simulink model "RoboBoatVU_2014_Athena"  (R2014a)
settings: Solver=FixedStepDiscrete  StartTime=0.0  StopTime=inf  FixedStep=.1  RelTol=1e-3
undefined symbols (not defined in the file): Com1, Com2, Com3, Com4, DiscIntNeverNeededParam, RGB24, standard, strel
libraries: visiontextngfix x25, dspmtrx3 x22, simulink x19, xpcseriallib x12, slrtlib x7, speedgoatlib_IO102 x6, dspstat3 x5, visionstatistics x3, dspindex x2, xpcvideousblib x2, xpcvideoutillib x2, visionmorphops x1
(part 1 of 4)
settings Model: BufferReuse=off  Creator=wildcat  LastModifiedBy=Villanova ASV
settings SolverCC: EnableConcurrentExecution=on
settings DataIOCC: SignalLoggingSaveFormat=ModelDataLogs
settings OptimizationCC: BlockReduction=off  OptimizeBlockIOStorage=off  BufferReuse=off  GlobalBufferReuse=off  ExpressionFolding=off  LocalBlockOutputs=off
settings DebuggingCC: UnderspecifiedInitializationDetection=Classic  StateNameClashWarn=warning
settings HardwareCC: ProdIntDivRoundTo=Zero  ProdEndianess=LittleEndian  ProdHWDeviceType=Generic->32-bit x86 compatible
settings RTWCC: SystemTargetFile=slrt.tlc  TemplateMakefile=slrt_default_tmf  Description=Simulink Real-Time  ProcessScript=slrt_make_rtw_hook  RTWCompilerOptimization=On
settings SimulinkRealTimeCC: GeneratePreprocessorConditionals=Disable all  EnableShiftOperators=on

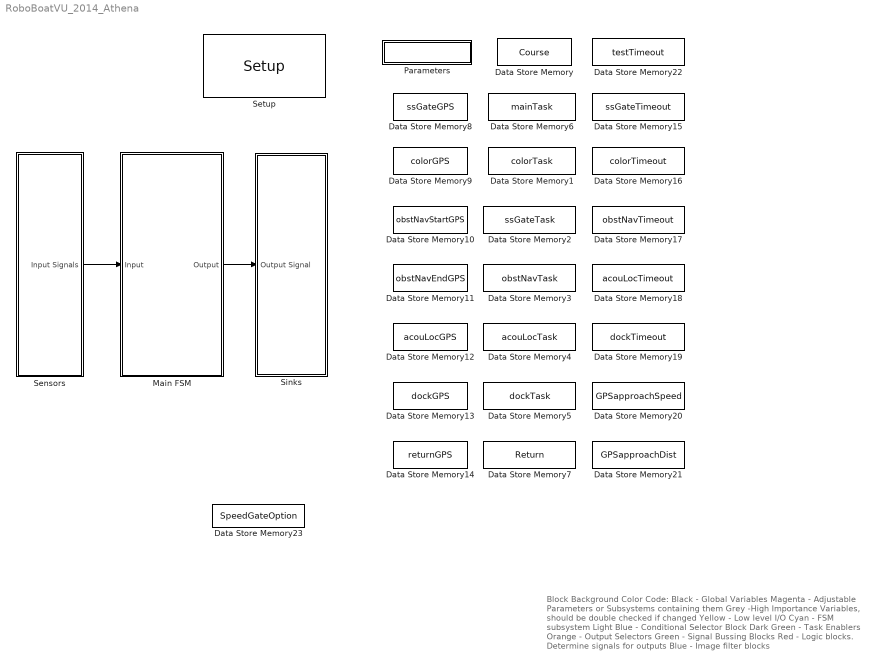
== system RoboBoatVU_2014_Athena ==
  note: Block Background Color Code:
      | Black - Global Variables
      | Magenta - Adjustable Parameters or Subsystems containing them
      | Grey -High Importance Variables, should be double checked if changed
      | Yellow - Low level I/O
      | Cyan - FSM subsystem
      | Light Blue - Conditional Selector Block
      | Dark Green - Task Enablers
      | Orange - Output Selectors
      | Green - Signal Bussing Blocks
      | Red - Logic blocks. Determine signals for outputs
      | Blue - Image filter blocks
  Data Store Memory : DataStoreMemory  DataStoreName=Course  ReadBeforeWriteMsg=warning  WriteAfterWriteMsg=warning  WriteAfterReadMsg=warning
  Data Store Memory1 : DataStoreMemory  DataStoreName=colorTask  ReadBeforeWriteMsg=warning  WriteAfterWriteMsg=warning  WriteAfterReadMsg=warning  InitialValue=zeros(1,8)
  Data Store Memory10 : DataStoreMemory  DataStoreName=obstNavStartGPS  ReadBeforeWriteMsg=warning  WriteAfterWriteMsg=warning  WriteAfterReadMsg=warning  InitialValue=zeros(1,2)
  Data Store Memory11 : DataStoreMemory  DataStoreName=obstNavEndGPS  ReadBeforeWriteMsg=warning  WriteAfterWriteMsg=warning  WriteAfterReadMsg=warning  InitialValue=zeros(1,2)
  Data Store Memory12 : DataStoreMemory  DataStoreName=acouLocGPS  ReadBeforeWriteMsg=warning  WriteAfterWriteMsg=warning  WriteAfterReadMsg=warning  InitialValue=zeros(1,2)
  Data Store Memory13 : DataStoreMemory  DataStoreName=dockGPS  ReadBeforeWriteMsg=warning  WriteAfterWriteMsg=warning  WriteAfterReadMsg=warning  InitialValue=zeros(1,2)
  Data Store Memory14 : DataStoreMemory  DataStoreName=returnGPS  ReadBeforeWriteMsg=warning  WriteAfterWriteMsg=warning  WriteAfterReadMsg=warning  InitialValue=zeros(1,2)
  Data Store Memory15 : DataStoreMemory  DataStoreName=ssGateTimeout  ReadBeforeWriteMsg=warning  WriteAfterWriteMsg=warning  WriteAfterReadMsg=warning
  Data Store Memory16 : DataStoreMemory  DataStoreName=colorTimeout  ReadBeforeWriteMsg=warning  WriteAfterWriteMsg=warning  WriteAfterReadMsg=warning
  Data Store Memory17 : DataStoreMemory  DataStoreName=obstNavTimeout  ReadBeforeWriteMsg=warning  WriteAfterWriteMsg=warning  WriteAfterReadMsg=warning
  Data Store Memory18 : DataStoreMemory  DataStoreName=acouLocTimeout  ReadBeforeWriteMsg=warning  WriteAfterWriteMsg=warning  WriteAfterReadMsg=warning
  Data Store Memory19 : DataStoreMemory  DataStoreName=dockTimeout  ReadBeforeWriteMsg=warning  WriteAfterWriteMsg=warning  WriteAfterReadMsg=warning
  Data Store Memory2 : DataStoreMemory  DataStoreName=ssGateTask  ReadBeforeWriteMsg=warning  WriteAfterWriteMsg=warning  WriteAfterReadMsg=warning  InitialValue=zeros(1,8)
  Data Store Memory20 : DataStoreMemory  DataStoreName=GPSapproachSpeed  ReadBeforeWriteMsg=warning  WriteAfterWriteMsg=warning  WriteAfterReadMsg=warning
  Data Store Memory21 : DataStoreMemory  DataStoreName=GPSapproachDist  ReadBeforeWriteMsg=warning  WriteAfterWriteMsg=warning  WriteAfterReadMsg=warning
  Data Store Memory22 : DataStoreMemory  DataStoreName=testTimeout  ReadBeforeWriteMsg=warning  WriteAfterWriteMsg=warning  WriteAfterReadMsg=warning
  Data Store Memory23 : DataStoreMemory  DataStoreName=SpeedGateOption  ReadBeforeWriteMsg=warning  WriteAfterWriteMsg=warning  WriteAfterReadMsg=warning  InitialValue=zeros(1,8)
  Data Store Memory3 : DataStoreMemory  DataStoreName=obstNavTask  ReadBeforeWriteMsg=warning  WriteAfterWriteMsg=warning  WriteAfterReadMsg=warning  InitialValue=zeros(1,8)
  Data Store Memory4 : DataStoreMemory  DataStoreName=acouLocTask  ReadBeforeWriteMsg=warning  WriteAfterWriteMsg=warning  WriteAfterReadMsg=warning  InitialValue=zeros(1,8)
  Data Store Memory5 : DataStoreMemory  DataStoreName=dockTask  ReadBeforeWriteMsg=warning  WriteAfterWriteMsg=warning  WriteAfterReadMsg=warning  InitialValue=zeros(1,8)
  Data Store Memory6 : DataStoreMemory  DataStoreName=mainTask  ReadBeforeWriteMsg=warning  WriteAfterWriteMsg=warning  WriteAfterReadMsg=warning  InitialValue=zeros(1,8)
  Data Store Memory7 : DataStoreMemory  DataStoreName=Return  ReadBeforeWriteMsg=warning  WriteAfterWriteMsg=warning  WriteAfterReadMsg=warning  InitialValue=zeros(1,8)
  Data Store Memory8 : DataStoreMemory  DataStoreName=ssGateGPS  ReadBeforeWriteMsg=warning  WriteAfterWriteMsg=warning  WriteAfterReadMsg=warning  InitialValue=zeros(1,2)
  Data Store Memory9 : DataStoreMemory  DataStoreName=colorGPS  ReadBeforeWriteMsg=warning  WriteAfterWriteMsg=warning  WriteAfterReadMsg=warning  InitialValue=zeros(1,2)
  Main FSM : Subsystem
  Parameters : Subsystem
  Sensors : Subsystem
  Setup : speedgoatlib_IO102/Setup  group=Digital output setup  id=1  range=+-5V  cal=off  pciSlot=-1  adChannelMode=Multiple-channel (enter number of channels below)  adChannel=16  adCoupling=Differential  daChannel=[1,2,3,4]  daReset=[1]  daInitValue=[0]  diChannel=[1,2,3,4,5,6,7,8]  doChannel=[1,2,3,4,5,6,7,8]  doReset=[1]  doInitValue=[0]
  Sinks : Subsystem
  wires:
  Main FSM/1(Output) -> Sinks/1(Output Signal)
  Sensors/1(Input Signals) -> Main FSM/1(Input)

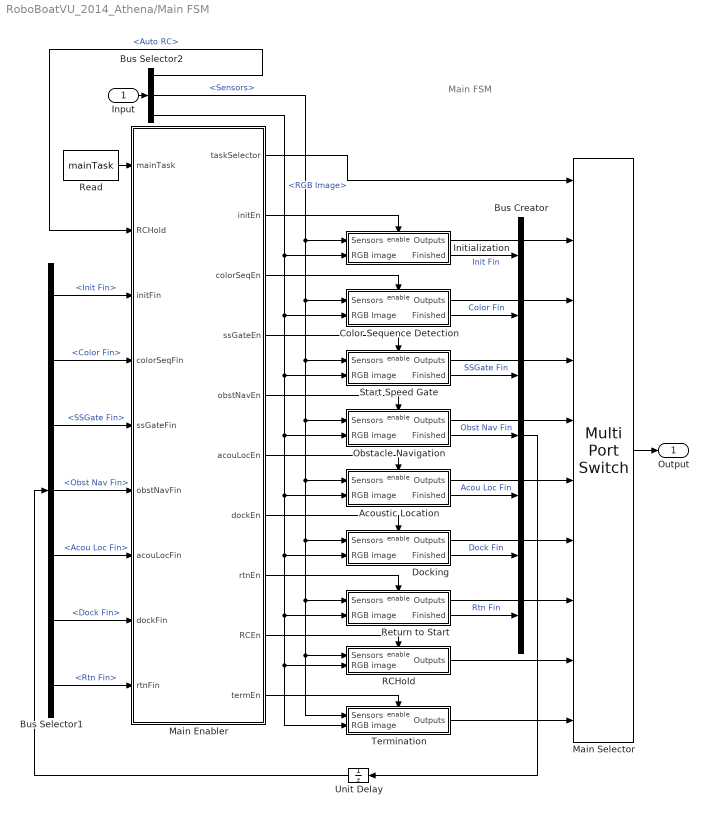
== system RoboBoatVU_2014_Athena/Main FSM ==
  note: Main FSM
  Input : Inport
  Acoustic Location : Subsystem  TreatAsAtomicUnit=on
  Bus Creator : BusCreator  Inputs=7
  Bus Selector1 : BusSelector  OutputSignals=Init Fin,Color Fin,SSGate Fin,Obst Nav Fin,Acou Loc Fin,Dock Fin,Rtn Fin
  Bus Selector2 : BusSelector  OutputSignals=Sensors.Digital In.Auto RC,Sensors,RGB Image
  Color Sequence Detection : Subsystem  TreatAsAtomicUnit=on
  Docking : Subsystem  TreatAsAtomicUnit=on
  Initialization : Subsystem
  Main Enabler : MATLAB Function  TreatAsAtomicUnit=on
  Main Selector : MultiPortSwitch  Inputs=9
  Obstacle Navigation : Subsystem  TreatAsAtomicUnit=on
  RCHold : Subsystem
  Read : DataStoreRead  DataStoreName=mainTask  SampleTime=0.1
  Return to Start : Subsystem  TreatAsAtomicUnit=on
  Start Speed Gate : Subsystem  TreatAsAtomicUnit=on
  Termination : Subsystem  TreatAsAtomicUnit=on
  Unit Delay : UnitDelay  SampleTime=-1
  Output : Outport
  wires:
  Bus Creator/1 -> Unit Delay/1
  Initialization/1(Outputs) -> Main Selector/2
  Main Selector/1 -> Output/1
  Read/1 -> Main Enabler/1(mainTask)
  Main Enabler/1(taskSelector) -> Main Selector/1
  Initialization/2(Finished) -> Bus Creator/1  "Init Fin"
  Unit Delay/1 -> Bus Selector1/1
  Input/1 -> Bus Selector2/1
  Bus Selector2/1 -> Main Enabler/2(RCHold)  "<Auto RC>"
  Main Enabler/2(initEn) -> Initialization/Enable
  Termination/1(Outputs) -> Main Selector/10
  RCHold/1(Outputs) -> Main Selector/9
  Main Enabler/9(RCEn) -> RCHold/Enable
  Main Enabler/10(termEn) -> Termination/Enable
  Bus Selector2/2 -> Initialization/1(Sensors), Color Sequence Detection/1(Sensors), Start Speed Gate/1(Sensors), Obstacle Navigation/1(Sensors), Docking/1(Sensors), Return to Start/1(Sensors), RCHold/1(Sensors), Termination/1(Sensors), Acoustic Location/1(Sensors)  "<Sensors>"
  Bus Selector2/3 -> Initialization/2(RGB image), Color Sequence Detection/2(RGB Image), Start Speed Gate/2(RGB image), Obstacle Navigation/2(RGB image), Docking/2(RGB image), Return to Start/2(RGB image), Termination/2(RGB image), RCHold/2(RGB image), Acoustic Location/2(RGB image)  "<RGB Image>"
  Color Sequence Detection/2(Finished) -> Bus Creator/2  "Color Fin"
  Start Speed Gate/2(Finished) -> Bus Creator/3  "SSGate Fin"
  Obstacle Navigation/2(Finished) -> Bus Creator/4  "Obst Nav Fin"
  Acoustic Location/2(Finished) -> Bus Creator/5  "Acou Loc Fin"
  Docking/2(Finished) -> Bus Creator/6  "Dock Fin"
  Return to Start/2(Finished) -> Bus Creator/7  "Rtn Fin"
  Return to Start/1(Outputs) -> Main Selector/8
  Docking/1(Outputs) -> Main Selector/7
  Acoustic Location/1(Outputs) -> Main Selector/6
  Obstacle Navigation/1(Outputs) -> Main Selector/5
  Start Speed Gate/1(Outputs) -> Main Selector/4
  Color Sequence Detection/1(Outputs) -> Main Selector/3
  Main Enabler/3(colorSeqEn) -> Color Sequence Detection/Enable
  Main Enabler/5(obstNavEn) -> Obstacle Navigation/Enable
  Main Enabler/6(acouLocEn) -> Acoustic Location/Enable
  Main Enabler/7(dockEn) -> Docking/Enable
  Main Enabler/8(rtnEn) -> Return to Start/Enable
  Bus Selector1/6 -> Main Enabler/8(dockFin)  "<Dock Fin>"
  Bus Selector1/1 -> Main Enabler/3(initFin)  "<Init Fin>"
  Bus Selector1/4 -> Main Enabler/6(obstNavFin)  "<Obst Nav Fin>"
  Bus Selector1/5 -> Main Enabler/7(acouLocFin)  "<Acou Loc Fin>"
  Bus Selector1/2 -> Main Enabler/4(colorSeqFin)  "<Color Fin>"
  Bus Selector1/3 -> Main Enabler/5(ssGateFin)  "<SSGate Fin>"
  Bus Selector1/7 -> Main Enabler/9(rtnFin)  "<Rtn Fin>"
  Main Enabler/4(ssGateEn) -> Start Speed Gate/Enable

== system RoboBoatVU_2014_Athena/Parameters ==
  note: Course options are:
      | A, B and
      | otherwise (for testing,
      |  must be one character)
  CourseName : Constant  Value=uint8('T')  VectorParams1D=off
  GPS Points : Subsystem
  Task Options : Subsystem
  Task Selector : Subsystem
  Timeouts and Constants : Subsystem
  Write : DataStoreWrite  DataStoreName=Course
  wires:
  CourseName/1 -> Write/1

== system RoboBoatVU_2014_Athena/Sensors ==
  Analog In : Subsystem
  Bus Creator : BusCreator  Inputs=2
  Bus Creator1 : BusCreator  Inputs=2
  Digital In : Subsystem
  Serial In : Subsystem
  Video In : Subsystem
  Input Signals : Outport
  wires:
  Serial In/1(Serial In) -> Bus Creator/1
  Digital In/1(Digital In) -> Bus Creator/2
  Video In/1(RGB image) -> Bus Creator1/2
  Bus Creator/1 -> Bus Creator1/1  "Sensors"
  Bus Creator1/1 -> Input Signals/1

== system RoboBoatVU_2014_Athena/Sinks ==
  Output Signal : Inport
  Bus Selector : BusSelector  OutputSignals=Sensors.Serial In.Compass.Heading,Outputs.Control Signals,Outputs.Annotated Image,Outputs.Control Signals.Arduino Signals
  Digital Outputs : Subsystem
  Image Transmission : Subsystem
  actuators : Subsystem
  data log : Subsystem  Commented=on
  wires:
  Bus Selector/2 -> actuators/2(Control Signals)  "<Control Signals>"
  Bus Selector/3 -> Image Transmission/1(RGB Image)  "<Annotated Image>"
  Bus Selector/1 -> actuators/1(Compass Heading)  "<Heading>"
  Output Signal/1 -> data log/1(Output signal), Bus Selector/1
  Bus Selector/4 -> Digital Outputs/1(Digital Outputs)  "<Arduino Signals>"

== system RoboBoatVU_2014_Athena/Main FSM/Acoustic Location ==
  note: Acoustic Location
  Sensors : Inport
  RGB image : Inport  Port=2
  Enable : EnablePort
  Bus Creator : BusCreator
  Bus Selector : BusSelector  OutputSignals=Mid S Fin,Left T Fin,Left S Fin,Right T Fin
  Bus Selector1 : BusSelector  OutputSignals=Output Signals,Task Finished
  Left Sample : Subsystem  TreatAsAtomicUnit=on
  Left Turn : Subsystem  TreatAsAtomicUnit=on
  MATLAB Function : MATLAB Function  TreatAsAtomicUnit=on
  Mid Sample : Subsystem  TreatAsAtomicUnit=on
  Multiport Switch : MultiPortSwitch  Inputs=5
  Right Sample : Subsystem  TreatAsAtomicUnit=on
  Right Turn : Subsystem  TreatAsAtomicUnit=on
  Unit Delay : UnitDelay  SampleTime=-1
  Outputs : Outport
  Finished : Outport  Port=2
  wires:
  Sensors/1 -> Left Turn/1(Sensors), Left Sample/1(Sensors), Right Turn/1(Sensors), Right Sample/1(Sensors), Mid Sample/1(Sensors)
  RGB image/1 -> Mid Sample/2(RGB Image), Left Turn/2(RGB Image), Right Turn/2(RGB Image), Right Sample/2(RGB Image), Left Sample/2(RGB Image)
  MATLAB Function/1(taskSelector) -> Multiport Switch/1
  MATLAB Function/2(midSampleEn) -> Mid Sample/Enable
  MATLAB Function/3(leftTurnEn) -> Left Turn/Enable
  MATLAB Function/4(leftSampleEn) -> Left Sample/Enable
  MATLAB Function/5(rightTurnEn) -> Right Turn/Enable
  MATLAB Function/6(rightSampleEn) -> Right Sample/Enable
  Mid Sample/1(Outputs) -> Multiport Switch/2
  Left Turn/1(Outputs) -> Multiport Switch/3
  Left Sample/1(Outputs) -> Multiport Switch/4
  Right Turn/1(Outputs) -> Multiport Switch/5
  Right Sample/1(Outputs) -> Multiport Switch/6
  Mid Sample/2(Finished) -> Bus Creator/1  "Mid S Fin"
  Left Turn/2(Finished) -> Bus Creator/2  "Left T Fin"
  Left Sample/2(Finished) -> Bus Creator/3  "Left S Fin"
  Right Turn/2(Finished) -> Bus Creator/4  "Right T Fin"
  Bus Creator/1 -> Unit Delay/1
  Unit Delay/1 -> Bus Selector/1
  Bus Selector/1 -> MATLAB Function/1(midSampleFin)  "<Mid S Fin>"
  Bus Selector/4 -> MATLAB Function/4(rightTurnFin)  "<Right T Fin>"
  Bus Selector/2 -> MATLAB Function/2(leftTurnFin)  "<Left T Fin>"
  Bus Selector/3 -> MATLAB Function/3(leftSampleFin)  "<Left S Fin>"
  Multiport Switch/1 -> Bus Selector1/1
  Bus Selector1/2 -> Finished/1  "<Task Finished>"
  Bus Selector1/1 -> Outputs/1  "<Output Signals>"

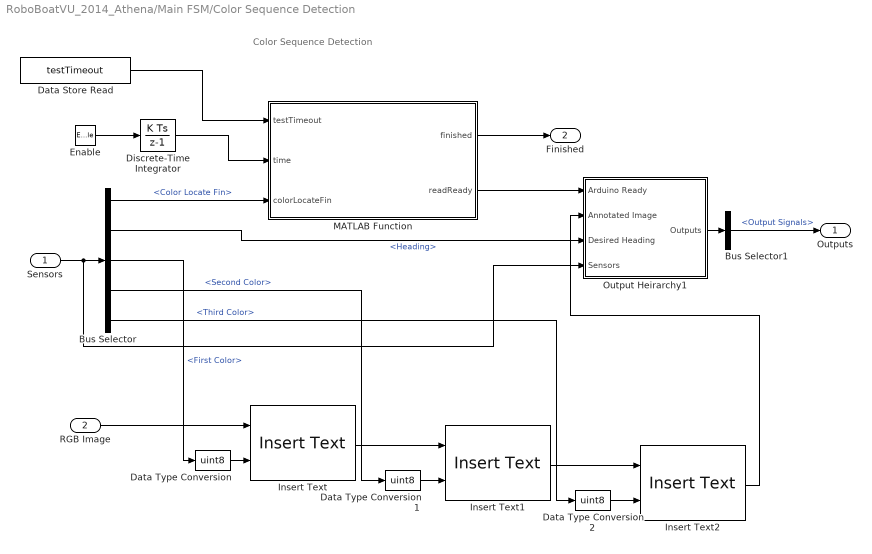
== system RoboBoatVU_2014_Athena/Main FSM/Color Sequence Detection ==
  note: Color Sequence Detection
  Sensors : Inport
  RGB Image : Inport  Port=2
  Enable : EnablePort  ShowOutputPort=on
  Bus Selector : BusSelector  OutputSignals=Digital In.Color Locate Fin,Serial In.Compass.Heading,Serial In.Arduino Messages.First Color,Serial In.Arduino Messages.Second Color,Serial In.Arduino Messages.Third Color
  Bus Selector1 : BusSelector  OutputSignals=Output Signals
  Data Store Read : DataStoreRead  DataStoreName=testTimeout
  Data Type Conversion : DataTypeConversion  OutDataTypeStr=uint8
  Data Type Conversion1 : DataTypeConversion  OutDataTypeStr=uint8
  Data Type Conversion2 : DataTypeConversion  OutDataTypeStr=uint8
  Discrete-Time Integrator : DiscreteIntegrator  SampleTime=0.1  ICPrevOutput=DiscIntNeverNeededParam  ICPrevScaledInput=DiscIntNeverNeededParam
  Insert Text : visiontextngfix/Insert Text  inputType=Obsolete  theText='First Color: %d'  getTextLocFrom=Specify via dialog  textLoc=[1 1]  getTextColorFrom=Specify via dialog  textColor=[0 0 0]  getTextIntensityFrom=Specify via dialog  textIntensity=0  getTextOpacityFrom=Specify via dialog  textOpacity=1.0  dummyVar2=0  dummyVar3=0  dummyVar4=0  imagePorts=One multidimensional signal  isInputTransposed=off  fontFace=LucidaSansRegular  dummyVar1=0  blockFontSize=12  antiAliased=on
  Insert Text1 : visiontextngfix/Insert Text  inputType=Obsolete  theText='Second Color: %d'  getTextLocFrom=Specify via dialog  textLoc=[1 10]  getTextColorFrom=Specify via dialog  textColor=[0 0 0]  getTextIntensityFrom=Specify via dialog  textIntensity=0  getTextOpacityFrom=Specify via dialog  textOpacity=1.0  dummyVar2=0  dummyVar3=0  dummyVar4=0  imagePorts=One multidimensional signal  isInputTransposed=off  fontFace=LucidaSansRegular  dummyVar1=0  blockFontSize=12  antiAliased=on
  Insert Text2 : visiontextngfix/Insert Text  inputType=Obsolete  theText='Third Color: %d'  getTextLocFrom=Specify via dialog  textLoc=[1 20]  getTextColorFrom=Specify via dialog  textColor=[0 0 0]  getTextIntensityFrom=Specify via dialog  textIntensity=0  getTextOpacityFrom=Specify via dialog  textOpacity=1.0  dummyVar2=0  dummyVar3=0  dummyVar4=0  imagePorts=One multidimensional signal  isInputTransposed=off  fontFace=LucidaSansRegular  dummyVar1=0  blockFontSize=12  antiAliased=on
  MATLAB Function : MATLAB Function  TreatAsAtomicUnit=on
  Output Heirarchy1 : Subsystem
  Outputs : Outport
  Finished : Outport  Port=2
  wires:
  Sensors/1 -> Output Heirarchy1/4(Sensors), Bus Selector/1
  Bus Selector/1 -> MATLAB Function/3(colorLocateFin)  "<Color Locate Fin>"
  MATLAB Function/2(readReady) -> Output Heirarchy1/1(Arduino Ready)
  RGB Image/1 -> Insert Text/1
  Bus Selector/3 -> Data Type Conversion/1  "<First Color>"
  Insert Text/1 -> Insert Text1/1
  Bus Selector/4 -> Data Type Conversion1/1  "<Second Color>"
  Insert Text1/1 -> Insert Text2/1
  Bus Selector/5 -> Data Type Conversion2/1  "<Third Color>"
  Bus Selector/2 -> Output Heirarchy1/3(Desired Heading)  "<Heading>"
  Insert Text2/1 -> Output Heirarchy1/2(Annotated Image)
  MATLAB Function/1(finished) -> Finished/1
  Enable/1 -> Discrete-Time Integrator/1
  Discrete-Time Integrator/1 -> MATLAB Function/2(time)
  Data Store Read/1 -> MATLAB Function/1(testTimeout)
  Output Heirarchy1/1(Outputs) -> Bus Selector1/1
  Bus Selector1/1 -> Outputs/1  "<Output Signals>"
  Data Type Conversion/1 -> Insert Text/2
  Data Type Conversion1/1 -> Insert Text1/2
  Data Type Conversion2/1 -> Insert Text2/2

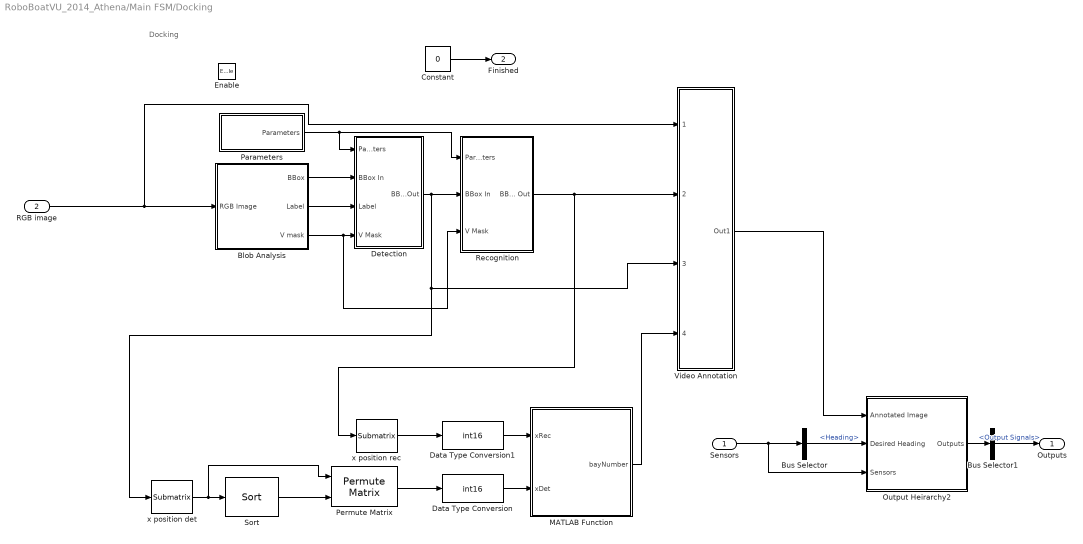
== system RoboBoatVU_2014_Athena/Main FSM/Docking ==
  note: Docking
  Sensors : Inport
  RGB image : Inport  Port=2
  Enable : EnablePort
  Blob Analysis : Subsystem
  Bus Selector : BusSelector  OutputSignals=Serial In.Compass.Heading
  Bus Selector1 : BusSelector  OutputSignals=Output Signals
  Constant : Constant  Value=0
  Data Type Conversion : DataTypeConversion  OutDataTypeStr=int16
  Data Type Conversion1 : DataTypeConversion  OutDataTypeStr=int16
  Detection : Subsystem
  MATLAB Function : MATLAB Function  TreatAsAtomicUnit=on
  Output Heirarchy2 : Subsystem
  Parameters : Subsystem
  Permute Matrix : dspmtrx3/Permute Matrix  mode=Rows  ZeroOneIdxMode=One-based  errmode=Clip index  checkDims=off
  Recognition : Subsystem
  Sort : dspstat3/Sort  otype=Index  dir=Ascending  sortAlg=Quick sort  accumDataTypeStr=Inherit: Same as product output  accumLastDataTypeStr=Inherit: Same as product output  roundingMode=Floor  overflowMode=off
  Video Annotation : Subsystem
  x position det : dspmtrx3/Submatrix  RowSpan=Range of rows  RowStartMode=First  RowStartIndex=1  RowEndMode=Last  RowEndIndex=1  ColSpan=One column  ColStartMode=First  ColStartIndex=1  ColEndMode=Last  ColEndIndex=1
  x position rec : dspmtrx3/Submatrix  RowSpan=Range of rows  RowStartMode=First  RowStartIndex=1  RowEndMode=Last  RowEndIndex=1  ColSpan=One column  ColStartMode=First  ColStartIndex=1  ColEndMode=Last  ColEndIndex=1
  Outputs : Outport
  Finished : Outport  Port=2
  wires:
  Blob Analysis/1("BBox ") -> Detection/2(BBox In)
  Blob Analysis/2(Label) -> Detection/3(Label)
  Parameters/1(Parameters) -> Recognition/1(Parameters), Detection/1(Parameters)
  Detection/1(BBox Out) -> Recognition/2(BBox In), x position det/1, Video Annotation/3(BBox Detect)
  Recognition/1(BBox Out) -> x position rec/1, Video Annotation/2(BBox Recognition)
  Blob Analysis/3(V mask) -> Recognition/3(V Mask), Detection/4(V Mask)
  x position det/1 -> Permute Matrix/1, Sort/1
  Sort/1 -> Permute Matrix/2
  x position rec/1 -> Data Type Conversion1/1
  Permute Matrix/1 -> Data Type Conversion/1
  MATLAB Function/1(bayNumber) -> Video Annotation/4(Bay Number)
  Data Type Conversion/1 -> MATLAB Function/2(xDet)
  Data Type Conversion1/1 -> MATLAB Function/1(xRec)
  RGB image/1 -> Blob Analysis/1(RGB Image), Video Annotation/1(RGB Image)
  Video Annotation/1(Out1) -> Output Heirarchy2/1(Annotated Image)
  Sensors/1 -> Output Heirarchy2/3(Sensors), Bus Selector/1
  Bus Selector/1 -> Output Heirarchy2/2(Desired Heading)  "<Heading>"
  Constant/1 -> Finished/1
  Output Heirarchy2/1(Outputs) -> Bus Selector1/1
  Bus Selector1/1 -> Outputs/1  "<Output Signals>"

== system RoboBoatVU_2014_Athena/Main FSM/Initialization ==
  Sensors : Inport
  RGB image : Inport  Port=2
  Enable : EnablePort
  Annotate Task : visiontextngfix/Insert Text  inputType=Obsolete  theText='Initializing...'  getTextLocFrom=Specify via dialog  textLoc=[10 10]  getTextColorFrom=Specify via dialog  textColor=[0 0 255]  getTextIntensityFrom=Specify via dialog  textIntensity=0  getTextOpacityFrom=Specify via dialog  textOpacity=1.0  dummyVar2=0  dummyVar3=0  dummyVar4=0  imagePorts=One multidimensional signal  isInputTransposed=off  fontFace=LucidaSansRegular  dummyVar1=0  blockFontSize=12  antiAliased=on
  Bus Selector : BusSelector  OutputSignals=Serial In.Compass.Heading
  Bus Selector1 : BusSelector  OutputSignals=Output Signals
  Output Heirarchy : Subsystem
  Wait 3 seconds : Step  Time=3  SampleTime=0
  Outputs : Outport
  Finished : Outport  Port=2
  wires:
  Sensors/1 -> Output Heirarchy/3(Sensors), Bus Selector/1  "Sensors"
  Bus Selector/1 -> Output Heirarchy/2(Desired Heading)  "<Heading>"
  RGB image/1 -> Annotate Task/1
  Annotate Task/1 -> Output Heirarchy/1(Annotated Image)
  Wait 3 seconds/1 -> Finished/1
  Output Heirarchy/1(Outputs) -> Bus Selector1/1
  Bus Selector1/1 -> Outputs/1  "<Output Signals>"

== system RoboBoatVU_2014_Athena/Main FSM/Obstacle Navigation ==
  note: Obstacle Navigation
  Sensors : Inport
  RGB image : Inport  Port=2
  Enable : EnablePort
  Bus Selector : BusSelector  OutputSignals=Serial In.Buoy Color,Serial In.Compass.Heading
  Bus Selector1 : BusSelector  OutputSignals=Output Signals
  Data Type Conversion : DataTypeConversion  OutDataTypeStr=uint8
  Insert Text : visiontextngfix/Insert Text  inputType=Obsolete  theText='Buoy Color: %d'  getTextLocFrom=Specify via dialog  textLoc=[1 1]  getTextColorFrom=Specify via dialog  textColor=[0 0 0]  getTextIntensityFrom=Specify via dialog  textIntensity=0  getTextOpacityFrom=Specify via dialog  textOpacity=1.0  dummyVar2=0  dummyVar3=0  dummyVar4=0  imagePorts=One multidimensional signal  isInputTransposed=off  fontFace=LucidaSansRegular  dummyVar1=0  blockFontSize=12  antiAliased=on
  Output Heirarchy1 : Subsystem
  Silly Action Decider : MATLAB Function  TreatAsAtomicUnit=on
  Outputs : Outport
  Finished : Outport  Port=2
  wires:
  Sensors/1 -> Output Heirarchy1/2(Sensors), Bus Selector/1  "Sensors"
  Silly Action Decider/2(finished) -> Finished/1
  Silly Action Decider/1(desiredHeading) -> Output Heirarchy1/1(Desired Heading)
  Bus Selector/1 -> Data Type Conversion/1, Silly Action Decider/1(buoyColor)  "<Buoy Color>"
  Bus Selector/2 -> Silly Action Decider/2(currentHeading)  "<Heading>"
  RGB image/1 -> Insert Text/1
  Insert Text/1 -> Output Heirarchy1/3(Annotated Image)
  Data Type Conversion/1 -> Insert Text/2
  Output Heirarchy1/1(Outputs) -> Bus Selector1/1
  Bus Selector1/1 -> Outputs/1  "<Output Signals>"

== system RoboBoatVU_2014_Athena/Main FSM/RCHold ==
  Sensors : Inport
  RGB image : Inport  Port=2
  Enable : EnablePort
  Annotate Task : visiontextngfix/Insert Text  inputType=Obsolete  theText='RC Hold'  getTextLocFrom=Specify via dialog  textLoc=[10 10]  getTextColorFrom=Specify via dialog  textColor=[0 0 255]  getTextIntensityFrom=Specify via dialog  textIntensity=0  getTextOpacityFrom=Specify via dialog  textOpacity=1.0  dummyVar2=0  dummyVar3=0  dummyVar4=0  imagePorts=One multidimensional signal  isInputTransposed=off  fontFace=LucidaSansRegular  dummyVar1=0  blockFontSize=12  antiAliased=on
  Bus Selector : BusSelector  OutputSignals=Serial In.Compass.Heading
  Bus Selector1 : BusSelector  OutputSignals=Output Signals
  Output Heirarchy1 : Subsystem
  Outputs : Outport
  wires:
  Sensors/1 -> Output Heirarchy1/3(Sensors), Bus Selector/1  "Sensors"
  Bus Selector/1 -> Output Heirarchy1/2(Desired Heading)  "<Heading>"
  RGB image/1 -> Annotate Task/1
  Annotate Task/1 -> Output Heirarchy1/1(Annotated Image)
  Output Heirarchy1/1(Outputs) -> Bus Selector1/1
  Bus Selector1/1 -> Outputs/1  "<Output Signals>"

== system RoboBoatVU_2014_Athena/Main FSM/Return to Start ==
  note: Return to Start
  Sensors : Inport
  RGB image : Inport  Port=2
  Enable : EnablePort  ShowOutputPort=on
  GPS: Center : Subsystem  TreatAsAtomicUnit=on
  Outputs : Outport
  Finished : Outport  Port=2
  wires:
  GPS: Center/1(Outputs) -> Outputs/1
  Sensors/1 -> GPS: Center/1(Sensors)  "Sensors"
  RGB image/1 -> GPS: Center/2(RGB image)
  Enable/1 -> GPS: Center/Enable
  GPS: Center/2(Finished) -> Finished/1

== system RoboBoatVU_2014_Athena/Main FSM/Start Speed Gate ==
  note: Start Speed Gate
  Sensors : Inport
  RGB image : Inport  Port=2
  Enable : EnablePort
  Data Store Read : DataStoreRead  DataStoreName=ssGateTask
  MATLAB Function : MATLAB Function  TreatAsAtomicUnit=on
  Multiport Switch : MultiPortSwitch  Inputs=2
  Start Speed Gate - Color : Subsystem  TreatAsAtomicUnit=on
  Start Speed Gate - LIDAR : Subsystem  TreatAsAtomicUnit=on
  Outputs : Outport
  Finished : Outport  Port=2
  wires:
  Data Store Read/1 -> MATLAB Function/1(SSGateTask)
  MATLAB Function/3(colorEn) -> Start Speed Gate - Color/Enable
  MATLAB Function/1(taskSelector) -> Multiport Switch/1
  RGB image/1 -> Start Speed Gate - LIDAR/2(RGB Image), Start Speed Gate - Color/2(RGB Image)
  Sensors/1 -> Start Speed Gate - LIDAR/1(Sensors), Start Speed Gate - Color/1(Sensors)  "Sensors"
  Start Speed Gate - Color/1(Outputs) -> Multiport Switch/3
  MATLAB Function/2(LIDAREn) -> Start Speed Gate - LIDAR/Enable
  Start Speed Gate - LIDAR/1(Output) -> Multiport Switch/2

== system RoboBoatVU_2014_Athena/Main FSM/Termination ==
  Sensors : Inport
  RGB image : Inport  Port=2
  Enable : EnablePort
  Annotate Task : visiontextngfix/Insert Text  inputType=Obsolete  theText='Terminating...'  getTextLocFrom=Specify via dialog  textLoc=[10 10]  getTextColorFrom=Specify via dialog  textColor=[0 0 255]  getTextIntensityFrom=Specify via dialog  textIntensity=0  getTextOpacityFrom=Specify via dialog  textOpacity=1.0  dummyVar2=0  dummyVar3=0  dummyVar4=0  imagePorts=One multidimensional signal  isInputTransposed=off  fontFace=LucidaSansRegular  dummyVar1=0  blockFontSize=12  antiAliased=on
  Bus Selector : BusSelector  OutputSignals=Serial In.Compass.Heading
  Bus Selector1 : BusSelector  OutputSignals=Output Signals
  Output Heirarchy1 : Subsystem
  Outputs : Outport
  wires:
  Sensors/1 -> Output Heirarchy1/3(Sensors), Bus Selector/1
  RGB image/1 -> Annotate Task/1
  Annotate Task/1 -> Output Heirarchy1/1(Annotated Image)  "Annotated Image"
  Bus Selector/1 -> Output Heirarchy1/2(Desired Heading)  "<Heading>"
  Output Heirarchy1/1(Outputs) -> Bus Selector1/1
  Bus Selector1/1 -> Outputs/1  "<Output Signals>"

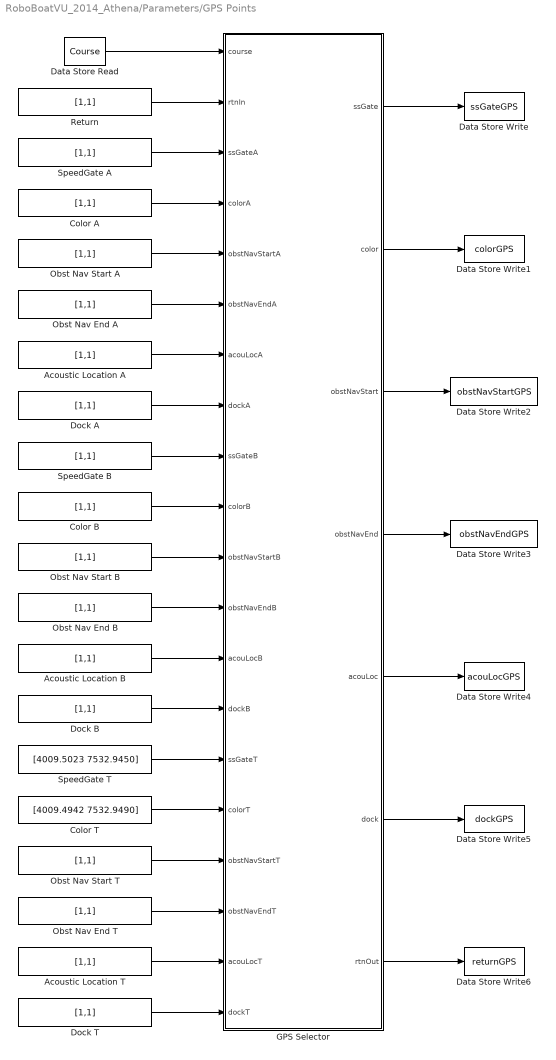
== system RoboBoatVU_2014_Athena/Parameters/GPS Points ==
  Acoustic Location A : Constant  Value=[1,1]  SampleTime=0.1
  Acoustic Location B : Constant  Value=[1,1]  SampleTime=0.1
  Acoustic Location T : Constant  Value=[1,1]  SampleTime=0.1
  Color A : Constant  Value=[1,1]  SampleTime=0.1
  Color B : Constant  Value=[1,1]  SampleTime=0.1
  Color T : Constant  Value=[4009.4942 7532.9490]  SampleTime=0.1
  Data Store Read : DataStoreRead  DialogController=Simulink.DDGSource  DataStoreName=Course  SampleTime=0.1
  Data Store Write : DataStoreWrite  DialogController=Simulink.DDGSource  DataStoreName=ssGateGPS
  Data Store Write1 : DataStoreWrite  DataStoreName=colorGPS
  Data Store Write2 : DataStoreWrite  DataStoreName=obstNavStartGPS
  Data Store Write3 : DataStoreWrite  DataStoreName=obstNavEndGPS
  Data Store Write4 : DataStoreWrite  DataStoreName=acouLocGPS
  Data Store Write5 : DataStoreWrite  DataStoreName=dockGPS
  Data Store Write6 : DataStoreWrite  DataStoreName=returnGPS
  Dock A : Constant  Value=[1,1]  SampleTime=0.1
  Dock B : Constant  Value=[1,1]  SampleTime=0.1
  Dock T : Constant  Value=[1,1]  SampleTime=0.1
  GPS Selector : MATLAB Function  TreatAsAtomicUnit=on
  Obst Nav End A : Constant  Value=[1,1]  SampleTime=0.1
  Obst Nav End B : Constant  Value=[1,1]  SampleTime=0.1
  Obst Nav End T : Constant  Value=[1,1]  SampleTime=0.1
  Obst Nav Start A : Constant  Value=[1,1]  SampleTime=0.1
  Obst Nav Start B : Constant  Value=[1,1]  SampleTime=0.1
  Obst Nav Start T : Constant  Value=[1,1]  SampleTime=0.1
  Return : Constant  Value=[1,1]  SampleTime=0.1
  SpeedGate A : Constant  Value=[1,1]  SampleTime=0.1
  SpeedGate B : Constant  Value=[1,1]  SampleTime=0.1
  SpeedGate T : Constant  Value=[4009.5023 7532.9450]  SampleTime=0.1
  wires:
  Data Store Read/1 -> GPS Selector/1(course)
  Return/1 -> GPS Selector/2(rtnIn)
  SpeedGate A/1 -> GPS Selector/3(ssGateA)
  Color A/1 -> GPS Selector/4(colorA)
  Obst Nav Start A/1 -> GPS Selector/5(obstNavStartA)
  Obst Nav End A/1 -> GPS Selector/6(obstNavEndA)
  SpeedGate T/1 -> GPS Selector/15(ssGateT)
  Acoustic Location T/1 -> GPS Selector/19(acouLocT)
  Color T/1 -> GPS Selector/16(colorT)
  Dock A/1 -> GPS Selector/8(dockA)
  Dock T/1 -> GPS Selector/20(dockT)
  Obst Nav End T/1 -> GPS Selector/18(obstNavEndT)
  Obst Nav Start T/1 -> GPS Selector/17(obstNavStartT)
  Obst Nav Start B/1 -> GPS Selector/11(obstNavStartB)
  Obst Nav End B/1 -> GPS Selector/12(obstNavEndB)
  Acoustic Location A/1 -> GPS Selector/7(acouLocA)
  Acoustic Location B/1 -> GPS Selector/13(acouLocB)
  Dock B/1 -> GPS Selector/14(dockB)
  SpeedGate B/1 -> GPS Selector/9(ssGateB)
  Color B/1 -> GPS Selector/10(colorB)
  GPS Selector/1(ssGate) -> Data Store Write/1
  GPS Selector/2(color) -> Data Store Write1/1
  GPS Selector/3(obstNavStart) -> Data Store Write2/1
  GPS Selector/4(obstNavEnd) -> Data Store Write3/1
  GPS Selector/5(acouLoc) -> Data Store Write4/1
  GPS Selector/6(dock) -> Data Store Write5/1
  GPS Selector/7(rtnOut) -> Data Store Write6/1

== system RoboBoatVU_2014_Athena/Parameters/Task Options ==
  note: otherwise skips and treats as buoys
  note: Options:
      | Shotgun
      | GPS
  note: *note*
      | left course generally has issues
      | treating the gates as buoys.
      | tends to find right course gates
      | and head towards them
  Fix length : MATLAB Function  TreatAsAtomicUnit=on
  Speed Gate Option : Constant  Value=uint8('Shotgun')
  Write : DataStoreWrite  DataStoreName=SpeedGateOption
  wires:
  Speed Gate Option/1 -> Fix length/1(selection)
  Fix length/1(adjusted) -> Write/1

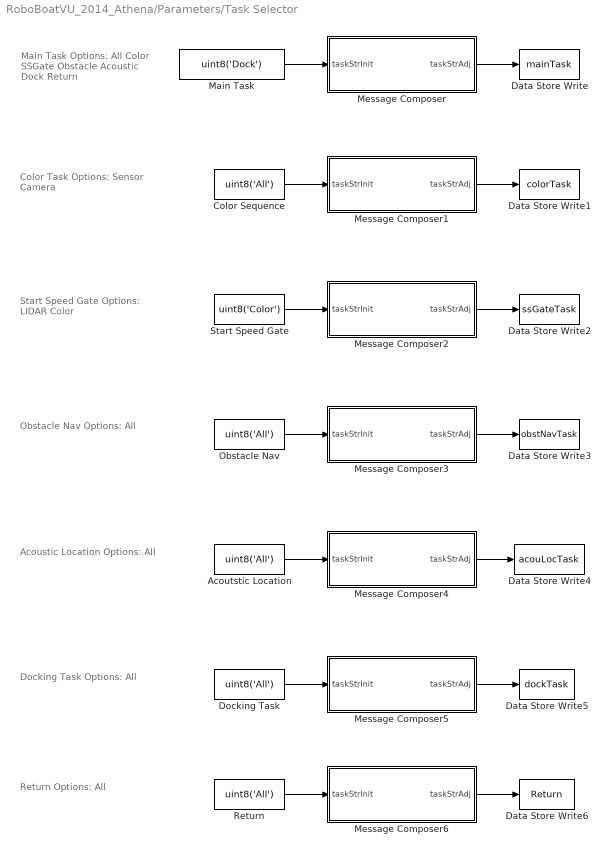
== system RoboBoatVU_2014_Athena/Parameters/Task Selector ==
  note: Docking Task Options:
      | All
  note: Acoustic Location Options:
      | All
  note: Obstacle Nav Options:
      | All
  note: Start Speed Gate Options:
      | LIDAR
      | Color
  note: Color Task Options:
      | Sensor
      | Camera
  note: Main Task Options:
      | All
      | Color
      | SSGate
      | Obstacle
      | Acoustic
      | Dock
      | Return
  note: Return Options:
      | All
  Acoutstic Location : Constant  Value=uint8('All')  SampleTime=0.1
  Color Sequence : Constant  Value=uint8('All')  SampleTime=0.1
  Data Store Write : DataStoreWrite  DataStoreName=mainTask
  Data Store Write1 : DataStoreWrite  DialogController=Simulink.DDGSource  DataStoreName=colorTask
  Data Store Write2 : DataStoreWrite  DataStoreName=ssGateTask
  Data Store Write3 : DataStoreWrite  DataStoreName=obstNavTask
  Data Store Write4 : DataStoreWrite  DataStoreName=acouLocTask
  Data Store Write5 : DataStoreWrite  DataStoreName=dockTask
  Data Store Write6 : DataStoreWrite  DataStoreName=Return
  Docking Task : Constant  Value=uint8('All')  SampleTime=0.1
  Main Task : Constant  Value=uint8('Dock')  SampleTime=0.1
  Message Composer : MATLAB Function  TreatAsAtomicUnit=on
  Message Composer1 : MATLAB Function  TreatAsAtomicUnit=on
  Message Composer2 : MATLAB Function  TreatAsAtomicUnit=on
  Message Composer3 : MATLAB Function  TreatAsAtomicUnit=on
  Message Composer4 : MATLAB Function  TreatAsAtomicUnit=on
  Message Composer5 : MATLAB Function  TreatAsAtomicUnit=on
  Message Composer6 : MATLAB Function  TreatAsAtomicUnit=on
  Obstacle Nav : Constant  Value=uint8('All')  SampleTime=0.1
  Return : Constant  Value=uint8('All')  SampleTime=0.1
  Start Speed Gate : Constant  Value=uint8('Color')  SampleTime=0.1
  wires:
  Main Task/1 -> Message Composer/1(taskStrInit)
  Message Composer/1(taskStrAdj) -> Data Store Write/1
  Color Sequence/1 -> Message Composer1/1(taskStrInit)
  Message Composer1/1(taskStrAdj) -> Data Store Write1/1
  Start Speed Gate/1 -> Message Composer2/1(taskStrInit)
  Message Composer2/1(taskStrAdj) -> Data Store Write2/1
  Obstacle Nav/1 -> Message Composer3/1(taskStrInit)
  Message Composer3/1(taskStrAdj) -> Data Store Write3/1
  Acoutstic Location/1 -> Message Composer4/1(taskStrInit)
  Message Composer4/1(taskStrAdj) -> Data Store Write4/1
  Docking Task/1 -> Message Composer5/1(taskStrInit)
  Message Composer5/1(taskStrAdj) -> Data Store Write5/1
  Return/1 -> Message Composer6/1(taskStrInit)
  Message Composer6/1(taskStrAdj) -> Data Store Write6/1

== system RoboBoatVU_2014_Athena/Parameters/Timeouts and Constants ==
  Acoustic Location Timeout : Constant  Value=30  SampleTime=0.1
  Color Timeout : Constant  Value=30  SampleTime=0.1
  Data Store Write : DataStoreWrite  DataStoreName=ssGateTimeout
  Data Store Write1 : DataStoreWrite  DataStoreName=colorTimeout
  Data Store Write2 : DataStoreWrite  DataStoreName=obstNavTimeout
  Data Store Write3 : DataStoreWrite  DataStoreName=acouLocTimeout
  Data Store Write4 : DataStoreWrite  DataStoreName=dockTimeout
  Data Store Write5 : DataStoreWrite  DataStoreName=GPSapproachSpeed
  Data Store Write6 : DataStoreWrite  DataStoreName=GPSapproachDist
  Data Store Write7 : DataStoreWrite  DataStoreName=testTimeout
  Docking Timeout : Constant  Value=30  SampleTime=0.1
  GPS Approach Distance : Constant  Value=3  SampleTime=0.1
  GPS Approach Speed : Constant  Value=4000  SampleTime=0.1
  Obstacle Nav Timeout : Constant  Value=30  SampleTime=0.1
  Start Speed Gate Timeout : Constant  Value=120  SampleTime=0.1
  Test Timeout : Constant  Value=15  SampleTime=0.1
  wires:
  Start Speed Gate Timeout/1 -> Data Store Write/1
  Color Timeout/1 -> Data Store Write1/1
  Acoustic Location Timeout/1 -> Data Store Write3/1
  Docking Timeout/1 -> Data Store Write4/1
  GPS Approach Speed/1 -> Data Store Write5/1
  GPS Approach Distance/1 -> Data Store Write6/1
  Obstacle Nav Timeout/1 -> Data Store Write2/1
  Test Timeout/1 -> Data Store Write7/1

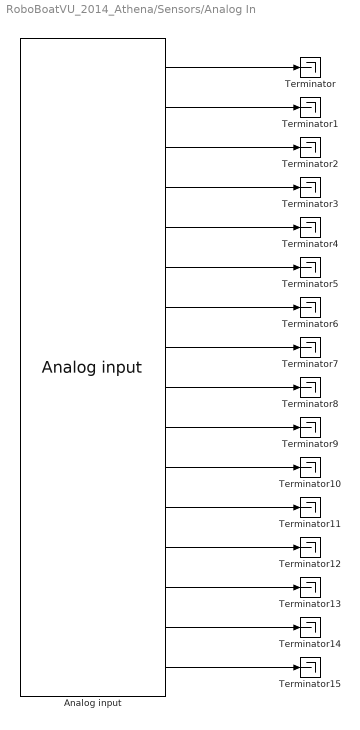
== system RoboBoatVU_2014_Athena/Sensors/Analog In ==
  Analog input : speedgoatlib_IO102/Analog input  id=1  channels=[1,2,3,4,5,6,7,8,9,10,11,12,13,14,15,16]  range=2  high_voltage=off  adCoupling=1  ts=0.1  pciSlot=-1
  Terminator{,1..15} (16 alike) : Terminator
  wires:
  Analog input/1 -> Terminator/1
  Analog input/2 -> Terminator1/1
  Analog input/3 -> Terminator2/1
  Analog input/4 -> Terminator3/1
  Analog input/5 -> Terminator4/1
  Analog input/6 -> Terminator5/1
  Analog input/7 -> Terminator6/1
  Analog input/8 -> Terminator7/1
  Analog input/9 -> Terminator8/1
  Analog input/10 -> Terminator9/1
  Analog input/11 -> Terminator10/1
  Analog input/12 -> Terminator11/1
  Analog input/13 -> Terminator12/1
  Analog input/14 -> Terminator13/1
  Analog input/15 -> Terminator14/1
  Analog input/16 -> Terminator15/1

== system RoboBoatVU_2014_Athena/Sensors/Digital In ==
  Bus Creator : BusCreator  Inputs=2
  Digital input : speedgoatlib_IO102/Digital input  id=1  channels=[1,2,3,4,5,6,7,8]  ts=0.1  pciSlot=-1
  Terminator{17..22} (6 alike) : Terminator
  Digital In : Outport
  wires:
  Bus Creator/1 -> Digital In/1  "Digital In"
  Digital input/8 -> Bus Creator/2  "Auto RC"
  Digital input/2 -> Terminator17/1
  Digital input/3 -> Terminator18/1
  Digital input/4 -> Terminator19/1
  Digital input/5 -> Terminator20/1
  Digital input/6 -> Terminator21/1
  Digital input/7 -> Terminator22/1
  Digital input/1 -> Bus Creator/1  "Color Locate Fin"

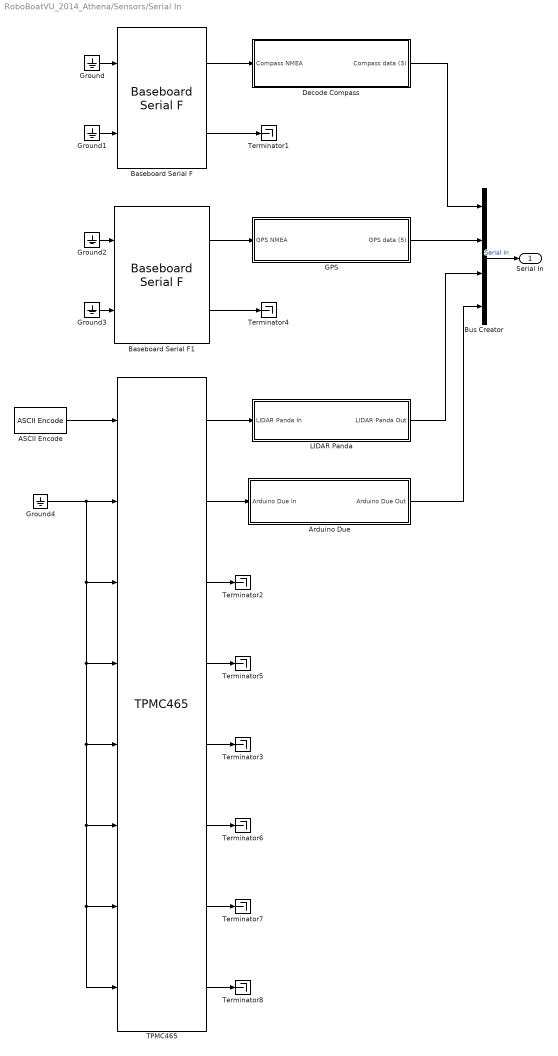
== system RoboBoatVU_2014_Athena/Sensors/Serial In ==
  " GPS" : Subsystem
  "ASCII Encode " : xpcseriallib/ASCII Encode   format=MSGS\r\n  nvars=0  maxlength=128  vartypes={ 'double' }
  Arduino Due : Subsystem
  Baseboard Serial F : xpcseriallib/Mainboard/Baseboard Serial F  group=Basic Setup  port=2  irqnum=4  saddr1=0x3f8  saddr2=0x3e8  config=Com1/Com3  baud1=19200  parity1=None  ndata1=8  nstop1=1  fifomode1=64 deep  rlevel1=half full  automode1=on  xmtfifosize1=1024  xmtdatatype1=8 bit uint null terminated  rcvfifosize1=1024  baud2=115200  parity2=None  ndata2=8  nstop2=1  fifomode2=64 deep  rlevel2=half full  automode2=on  xmtfifosize2=1024  xmtdatatype2=8 bit uint null terminated  rcvfifosize2=1024
  Baseboard Serial F1 : xpcseriallib/Mainboard/Baseboard Serial F  group=Basic Setup  port=2  irqnum=4  saddr1=0x3f8  saddr2=0x3e8  config=Com2/Com4  baud1=19200  parity1=None  ndata1=8  nstop1=1  fifomode1=64 deep  rlevel1=half full  automode1=on  xmtfifosize1=1024  xmtdatatype1=8 bit uint null terminated  rcvfifosize1=1024  baud2=115200  parity2=None  ndata2=8  nstop2=1  fifomode2=64 deep  rlevel2=half full  automode2=on  xmtfifosize2=1024  xmtdatatype2=8 bit uint null terminated  rcvfifosize2=1024
  Bus Creator : BusCreator
  Decode Compass : Subsystem
  Ground{,1..4} (5 alike) : Ground
  LIDAR Panda : Subsystem
  TPMC465 : speedgoatlib/IO504/TPMC465  group=Basic Setup  port=1  irqnum=9  slot=-1  transceiver1=RS232 (max 921.6kb/s)  standard1=on  baud1=115200  bauddivisor1=1  sampling1=16x (standard)  prescale1=off  parity1=None  ndata1=8  nstop1=1  rlevel1=half full (32)  hwmode1=none  swmode1=none  xonchar1=17  xoffchar1=19  rs485auto1=off  rs485delay1=0  xmtfifosize1=1024  xmtdatatype1=8 bit uint null terminated  rcvfifosize1=1024  transceiver2=RS232 (max 921.6kb/s)  standard2=on  baud2=115200  bauddivisor2=1  sampling2=16x (standard)  prescale2=off  parity2=None  ndata2=8  nstop2=1  rlevel2=half full (32)  hwmode2=none  swmode2=none  xonchar2=17  xoffchar2=19  rs485auto2=off  rs485delay2=0  xmtfifosize2=1024  xmtdatatype2=8 bit uint null terminated  rcvfifosize2=1024  transceiver3=RS232 (max 921.6kb/s)  standard3=on  baud3=115200  bauddivisor3=1  sampling3=16x (standard)  prescale3=off  parity3=None  ndata3=8  nstop3=1  rlevel3=half full (32)  hwmode3=none  swmode3=none  xonchar3=17  xoffchar3=19  rs485auto3=off  rs485delay3=0  xmtfifosize3=1024  xmtdatatype3=8 bit uint null terminated  rcvfifosize3=1024  transceiver4=RS232 (max 921.6kb/s)  standard4=on  baud4=115200  bauddivisor4=1  sampling4=16x (standard)  prescale4=off  parity4=None  ndata4=8  nstop4=1  rlevel4=half full (32)  hwmode4=none  swmode4=none  xonchar4=17  xoffchar4=19  rs485auto4=off  rs485delay4=0  xmtfifosize4=1024  xmtdatatype4=8 bit uint null terminated  rcvfifosize4=1024  transceiver5=RS232 (max 921.6kb/s)  standard5=on  baud5=115200  bauddivisor5=1  sampling5=16x (standard)  prescale5=off  parity5=None  ndata5=8  nstop5=1  rlevel5=1  hwmode5=none  swmode5=none  xonchar5=17  xoffchar5=19  rs485auto5=off  rs485delay5=0  xmtfifosize5=1024  xmtdatatype5=8 bit uint null terminated  rcvfifosize5=1024  transceiver6=RS232 (max 921.6kb/s)  standard6=on  baud6=115200  bauddivisor6=1  sampling6=16x (standard)  prescale6=off  parity6=None  ndata6=8  nstop6=1  rlevel6=1  hwmode6=none  swmode6=none  xonchar6=17  xoffchar6=19  rs485auto6=off  rs485delay6=0  xmtfifosize6=1024  xmtdatatype6=8 bit uint null terminated  rcvfifosize6=1024  transceiver7=RS232 (max 921.6kb/s)  standard7=on  baud7=115200  bauddivisor7=1  sampling7=16x (standard)  prescale7=off  parity7=None  ndata7=8  nstop7=1  rlevel7=1  hwmode7=none  swmode7=none  xonchar7=17  xoffchar7=19  rs485auto7=off  rs485delay7=0  xmtfifosize7=1024  xmtdatatype7=8 bit uint null terminated  rcvfifosize7=1024  transceiver8=RS232 (max 921.6kb/s)  standard8=on  baud8=115200  bauddivisor8=1  sampling8=16x (standard)  prescale8=off  parity8=None  ndata8=8  nstop8=1  rlevel8=1  hwmode8=none  swmode8=none  xonchar8=17  xoffchar8=19  rs485auto8=off  rs485delay8=0  xmtfifosize8=1024  xmtdatatype8=8 bit uint null terminated  rcvfifosize8=1024
  Terminator{1..8} (8 alike) : Terminator
  Serial In : Outport
  wires:
  Decode Compass/1(Compass data (3)) -> Bus Creator/1
  " GPS"/1(GPS data (5)) -> Bus Creator/2
  Bus Creator/1 -> Serial In/1  "Serial In"
  Ground4/1 -> TPMC465/3, TPMC465/6, TPMC465/8, TPMC465/7, TPMC465/5, TPMC465/4, TPMC465/2
  TPMC465/6 -> Terminator6/1
  TPMC465/7 -> Terminator7/1
  TPMC465/8 -> Terminator8/1
  TPMC465/5 -> Terminator3/1
  LIDAR Panda/1(LIDAR Panda Out) -> Bus Creator/3
  Ground/1 -> Baseboard Serial F/1
  Ground1/1 -> Baseboard Serial F/2
  Baseboard Serial F/1 -> Decode Compass/1(Compass NMEA)
  Ground3/1 -> Baseboard Serial F1/2
  Ground2/1 -> Baseboard Serial F1/1
  Baseboard Serial F1/1 -> " GPS"/1(GPS NMEA)
  Baseboard Serial F/2 -> Terminator1/1
  Baseboard Serial F1/2 -> Terminator4/1
  Arduino Due/1(Arduino Due Out) -> Bus Creator/4
  TPMC465/4 -> Terminator5/1
  TPMC465/3 -> Terminator2/1
  TPMC465/1 -> LIDAR Panda/1(LIDAR Panda In)
  TPMC465/2 -> Arduino Due/1(Arduino Due In)
  "ASCII Encode "/1 -> TPMC465/1

== system RoboBoatVU_2014_Athena/Sensors/Video In ==
  Constant : Constant  Commented=on  Value=uint8(255*ones(480,640,3))
  From USB Video Device : xpcvideousblib/From USB Video Device  sconf=<Select a configuration>  paddr=-1  iwidth=640  iheight=480  fint=1/10  ffmt=Uncompressed  cfmt=RGB24 (8:8:8)  isig=One multidimensional signal  trigger=off  status=off  updateBlock=1
  USB Video Device List : xpcvideousblib/USB Video Device List  usb_search=on  ShowInLibBrowser=0
  RGB image : Outport
  wires:
  From USB Video Device/1 -> RGB image/1  "RGB Image"

== system RoboBoatVU_2014_Athena/Sinks/Digital Outputs ==
  Digital Outputs : Inport
  Bus Selector : BusSelector  OutputSignals=Ready to Read,Due Sample Start
  Digital output : speedgoatlib_IO102/Digital output  id=1  channels=[1,2,3,4,5,6,7,8]  ts=0.1  pciSlot=-1
  Ground : Ground
  wires:
  Digital Outputs/1 -> Bus Selector/1
  Bus Selector/1 -> Digital output/1  "<Ready to Read>"
  Bus Selector/2 -> Digital output/2  "<Due Sample Start>"
  Ground/1 -> Digital output/4, Digital output/8, Digital output/7, Digital output/6, Digital output/5, Digital output/3

== system RoboBoatVU_2014_Athena/Sinks/Image Transmission ==
  note: Image Transmission
  RGB Image : Inport
  Image Transmit : xpcvideoutillib/Image Transmit  ipAddress=255.255.255.255  ipPort=25000  localPort=-1  vblLen=on  maxpacket=40*1024  sampletime=-1
  Jpeg Compression1 : xpcvideoutillib/Jpeg Compression  quality=20  cspace=RGB  isig=One multidimensional signal  maxsize=640*480  length=on
  Rate Transition : RateTransition  OutPortSampleTime=1
  wires:
  Jpeg Compression1/1 -> Image Transmit/1
  Jpeg Compression1/2 -> Image Transmit/2
  Rate Transition/1 -> Jpeg Compression1/1
  RGB Image/1 -> Rate Transition/1

== system RoboBoatVU_2014_Athena/Sinks/actuators ==
  Compass Heading : Inport
  Control Signals : Inport  Port=2
  analog output : Subsystem
  digital output : Subsystem
  wires:
  Control Signals/1 -> digital output/1(Digital Out), analog output/2(Control Signals)
  Compass Heading/1 -> analog output/1(Compass Heading)

== system RoboBoatVU_2014_Athena/Sinks/data log ==
  note: need to play with the boat to figure out how this works properly
  Output signal : Inport
  "Scope " : slrtlib/Displays and Logging/Scope   scopeno=1  scopetype=File  autostart=on  viewmode=Graphical redraw  formatstr='%15.6f'  grid=on  ylimits=[0,0]  nosamples=250  noprepostsamples=0  interleave=1  triggermode=Signal triggering  triggersignal=1  trigsignalfromport=on  triggerlevel=1  triggerslope=Rising  triggerscope=1  triggersample=0  filename=data.dat  mode=Lazy  writesize=512  autorestart=off  dynamicfilemode=off  maxwritefilesize=512*1024^2
  wires:
  Output signal/1 -> ?

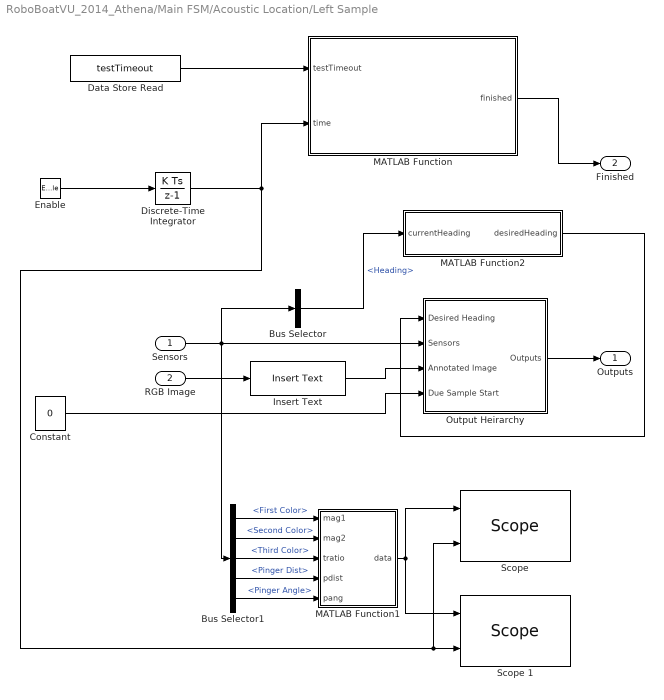
== system RoboBoatVU_2014_Athena/Main FSM/Acoustic Location/Left Sample ==
  Sensors : Inport
  RGB Image : Inport  Port=2
  Enable : EnablePort  ShowOutputPort=on
  Bus Selector : BusSelector  OutputSignals=Serial In.Compass.Heading
  Bus Selector1 : BusSelector  OutputSignals=Serial In.Arduino Messages.First Color,Serial In.Arduino Messages.Second Color,Serial In.Arduino Messages.Third Color,Serial In.Arduino Messages.Pinger Dist,Serial In.Arduino Messages.Pinger Angle
  Constant : Constant  Value=0  VectorParams1D=off
  Data Store Read : DataStoreRead  DataStoreName=testTimeout
  Discrete-Time Integrator : DiscreteIntegrator  SampleTime=0.1  ICPrevOutput=DiscIntNeverNeededParam  ICPrevScaledInput=DiscIntNeverNeededParam
  Insert Text : visiontextngfix/Insert Text  inputType=Obsolete  theText='Left Sample'  getTextLocFrom=Specify via dialog  textLoc=[1 1]  getTextColorFrom=Specify via dialog  textColor=[0 0 0]  getTextIntensityFrom=Specify via dialog  textIntensity=0  getTextOpacityFrom=Specify via dialog  textOpacity=1.0  dummyVar2=0  dummyVar3=0  dummyVar4=0  imagePorts=One multidimensional signal  isInputTransposed=off  fontFace=LucidaSansRegular  dummyVar1=0  blockFontSize=12  antiAliased=on
  MATLAB Function : MATLAB Function  TreatAsAtomicUnit=on
  MATLAB Function1 : MATLAB Function  TreatAsAtomicUnit=on
  MATLAB Function2 : MATLAB Function  TreatAsAtomicUnit=on
  Output Heirarchy : Subsystem
  "Scope " : slrtlib/Displays and Logging/Scope   scopeno=4  scopetype=File  autostart=on  viewmode=Graphical redraw  formatstr='%15.6f'  grid=on  ylimits=[0,0]  nosamples=100  noprepostsamples=0  interleave=1  triggermode=Signal triggering  triggersignal=1  trigsignalfromport=on  triggerlevel=1  triggerslope=Either  triggerscope=1  triggersample=0  filename=lsample2.dat  mode=Lazy  writesize=512  autorestart=off  dynamicfilemode=off  maxwritefilesize=512*1024^2
  Scope 1 : slrtlib/Displays and Logging/Scope   scopeno=5  scopetype=Host  autostart=on  viewmode=Graphical redraw  formatstr='%15.6f'  grid=on  ylimits=[0,0]  nosamples=100  noprepostsamples=0  interleave=1  triggermode=Signal triggering  triggersignal=1  trigsignalfromport=on  triggerlevel=1  triggerslope=Either  triggerscope=1  triggersample=0  filename=msample1.dat  mode=Lazy  writesize=512  autorestart=off  dynamicfilemode=off  maxwritefilesize=512*1024^2
  Outputs : Outport
  Finished : Outport  Port=2
  wires:
  RGB Image/1 -> Insert Text/1
  Insert Text/1 -> Output Heirarchy/3(Annotated Image)
  Bus Selector/1 -> MATLAB Function2/1(currentHeading)  "<Heading>"
  Output Heirarchy/1(Outputs) -> Outputs/1
  Data Store Read/1 -> MATLAB Function/1(testTimeout)
  MATLAB Function/1(finished) -> Finished/1
  Enable/1 -> Discrete-Time Integrator/1
  Sensors/1 -> Bus Selector1/1, Output Heirarchy/2(Sensors), Bus Selector/1
  Bus Selector1/5 -> MATLAB Function1/5(pang)  "<Pinger Angle>"
  Bus Selector1/2 -> MATLAB Function1/2(mag2)  "<Second Color>"
  Bus Selector1/1 -> MATLAB Function1/1(mag1)  "<First Color>"
  Bus Selector1/3 -> MATLAB Function1/3(tratio)  "<Third Color>"
  Bus Selector1/4 -> MATLAB Function1/4(pdist)  "<Pinger Dist>"
  MATLAB Function1/1(data) -> Scope 1/1, "Scope "/1
  Constant/1 -> Output Heirarchy/4(Due Sample Start)
  Discrete-Time Integrator/1 -> Scope 1/2, "Scope "/2, MATLAB Function/2(time)
  MATLAB Function2/1(desiredHeading) -> Output Heirarchy/1(Desired Heading)

== system RoboBoatVU_2014_Athena/Main FSM/Acoustic Location/Left Turn ==
  Sensors : Inport
  RGB Image : Inport  Port=2
  Enable : EnablePort
  Bus Selector : BusSelector  OutputSignals=Serial In.Compass.Heading
  Constant : Constant  Commented=on
  Insert Text : visiontextngfix/Insert Text  inputType=Obsolete  theText='Left Turn'  getTextLocFrom=Specify via dialog  textLoc=[1 1]  getTextColorFrom=Specify via dialog  textColor=[0 0 0]  getTextIntensityFrom=Specify via dialog  textIntensity=0  getTextOpacityFrom=Specify via dialog  textOpacity=1.0  dummyVar2=0  dummyVar3=0  dummyVar4=0  imagePorts=One multidimensional signal  isInputTransposed=off  fontFace=LucidaSansRegular  dummyVar1=0  blockFontSize=12  antiAliased=on
  Left Turn : MATLAB Function  TreatAsAtomicUnit=on
  Output Heirarchy : Subsystem
  Outputs : Outport
  Finished : Outport  Port=2
  wires:
  Sensors/1 -> Output Heirarchy/2(Sensors), Bus Selector/1
  Bus Selector/1 -> Left Turn/1(currentHeading)  "<Heading>"
  Left Turn/1(desiredHeading) -> Output Heirarchy/1(Desired Heading)
  RGB Image/1 -> Insert Text/1
  Insert Text/1 -> Output Heirarchy/3(Annotated Image)
  Output Heirarchy/1(Outputs) -> Outputs/1
  Left Turn/2(finished) -> Finished/1

== matlab function RoboBoatVU_2014_Athena/Main FSM/Acoustic Location/Mid Sample/MATLAB Function1 ==
  data: mag1 input; data output; mag2 input; tratio input; pdist input; pang input
function data = dataFormat(mag1,mag2,tratio,pdist,pang)

data = [mag1 mag2 tratio pdist pang];

== matlab function RoboBoatVU_2014_Athena/Main FSM/Acoustic Location/Left Sample/MATLAB Function1 ==
  data: mag1 input; data output; mag2 input; tratio input; pdist input; pang input
function data = dataFormat(mag1,mag2,tratio,pdist,pang)

data = [mag1 mag2 tratio pdist pang];

== matlab function RoboBoatVU_2014_Athena/Main FSM/Acoustic Location/Right Sample/MATLAB Function1 ==
  data: mag1 input; data output; mag2 input; tratio input; pdist input; pang input
function data = dataFormat(mag1,mag2,tratio,pdist,pang)

data = [mag1 mag2 tratio pdist pang];

== matlab function RoboBoatVU_2014_Athena/Main FSM/Start Speed Gate/MATLAB Function ==
  data: taskSelector output; SSGateTask input; LIDAREn output; colorEn output
function [taskSelector,LIDAREn,colorEn] = taskApproach(SSGateTask)

LIDAREn = 0;
colorEn = 0;

taskApproachStr = char(SSGateTask');

if ~isempty(strfind(taskApproachStr,'LIDAR'))
    LIDAREn = 1;
    taskSelector = 1;
elseif ~isempty(strfind(taskApproachStr,'Color'))
    colorEn = 1;
    taskSelector = 2;
end
